simulink model "Diagrama de blocos - Matlab-SimulinkArquivo"  (R2019a)
settings: Solver=VariableStepAuto  StartTime=0.0  StopTime=15  RelTol=1e-6
libraries: simulink x1
settings Model: Creator=rcard  LastModifiedBy=rcard

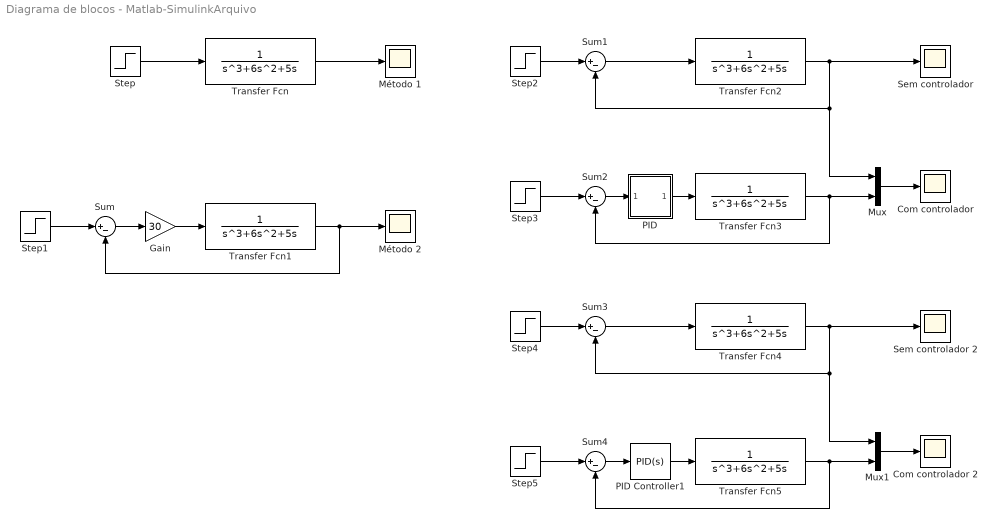
== system Diagrama de blocos - Matlab-SimulinkArquivo ==
  Com controlador : Scope
  Com controlador 2 : Scope
  Gain : Gain  Gain=30
  Mux : Mux  Inputs=2
  Mux1 : Mux  Inputs=2
  Método 1 : Scope
  Método 2 : Scope
  PID : Subsystem
  PID Controller1 : simulink/Continuous/PID Controller  Controller=PID  Form=Parallel  TimeDomain=Continuous-time  SampleTime=-1  IntegratorMethod=Forward Euler  FilterMethod=Forward Euler  ControllerParametersSource=internal  P=32.5  I=10.56  D=25  UseFilter=on  N=1000  TunerSelectOption=Transfer Function Based (PID Tuner App)  InitialConditionSource=internal  InitialConditionForIntegrator=0  InitialConditionForFilter=0  DifferentiatorICPrevScaledInput=0  ExternalReset=none  TrackingMode=off  Kt=1  LimitOutput=off  UpperSaturationLimit=inf  LowerSaturationLimit=-inf  LinearizeAsGain=on  AntiWindupMode=none  Kb=1  POutMin=[]  POutMax=[]  IOutMin=[]  IOutMax=[]  DOutMin=[]  DOutMax=[]  NOutMin=[]  NOutMax=[]  SumOutMin=[]  SumOutMax=[]  SaturationOutMin=[]  SaturationOutMax=[]  PParamMin=[]  PParamMax=[]  IParamMin=[]  IParamMax=[]  DParamMin=[]  DParamMax=[]  NParamMin=[]  NParamMax=[]  KbParamMin=[]  KbParamMax=[]  KtParamMin=[]  KtParamMax=[]  KbOutMin=[]  KbOutMax=[]  KtOutMin=[]  KtOutMax=[]  IntegratorOutMin=[]  IntegratorOutMax=[]  FilterOutMin=[]  FilterOutMax=[]  SumI1OutMin=[]  SumI1OutMax=[]  SumI2OutMin=[]  SumI2OutMax=[]  SumI3OutMin=[]  SumI3OutMax=[]  SumI4OutMin=[]  SumI4OutMax=[]  SumDOutMin=[]  SumDOutMax=[]  DifferentiatorOutMin=[]  DifferentiatorOutMax=[]  FilterDiffOutCoefMin=[]  FilterDiffOutCoefMax=[]  ReciprocalOutMin=[]  ReciprocalOutMax=[]  SumDenOutMin=[]  SumDenOutMax=[]  SumNumOutMin=[]  SumNumOutMax=[]  DivideOutMin=[]  DivideOutMax=[]  IntegratorContinuousStateAttributes=''  IntegratorStateMustResolveToSignalObject=off  IntegratorRTWStateStorageClass=Auto  FilterContinuousStateAttributes=''  FilterStateMustResolveToSignalObject=off  FilterRTWStateStorageClass=Auto  ParallelPVariant=InternalParameters  IdealPVariant=Disabled  IVariant=InternalParameters  DVariant=InternalParameters  IntegratorVariant=Continuous  SatVariant=Disabled  AWVariant=Passthrough  PCopyVariant=Disabled  TRVariant=Disabled  FdbkBlocksVariant=Forward  IdealPFdbkVariant=Disabled  SatFdbkVariant=Disabled  DerivativeFilterVariant=ContFilter  NVariant=InternalParameters  NCopyVariant=Disabled  FilterICVariant=InternalICsFilter  IntegratorICVariant=InternalICs  ExternalResetVariant=Disabled  TRSumVariant=Passthrough  SumFdbkVariant=Disabled  SumVariant=Sum_PID
  Sem controlador : Scope
  Sem controlador 2 : Scope
  Step{,1..5} (6 alike) : Step  Time=0  SampleTime=0
  Sum{,1..4} (5 alike) : Sum  Inputs=|+-
  Transfer Fcn{,1..5} (6 alike) : TransferFcn  Denominator="[1 6  5  0]"
  wires:
  Step1/1 -> Sum/1
  Sum/1 -> Gain/1
  Gain/1 -> Transfer Fcn1/1
  Transfer Fcn1/1 -> Sum/2, Método 2/1
  Transfer Fcn/1 -> Método 1/1
  Step/1 -> Transfer Fcn/1
  Step2/1 -> Sum1/1
  Transfer Fcn2/1 -> Mux/1, Sum1/2, Sem controlador/1
  Sum1/1 -> Transfer Fcn2/1
  Transfer Fcn3/1 -> Mux/2, Sum2/2
  Step3/1 -> Sum2/1
  Sum2/1 -> PID/1(In1)
  PID/1(Out1) -> Transfer Fcn3/1
  Mux/1 -> Com controlador/1
  Transfer Fcn4/1 -> Mux1/1, Sum3/2, Sem controlador 2/1
  Step5/1 -> Sum4/1
  Transfer Fcn5/1 -> Mux1/2, Sum4/2
  Sum3/1 -> Transfer Fcn4/1
  Mux1/1 -> Com controlador 2/1
  Sum4/1 -> PID Controller1/1
  PID Controller1/1 -> Transfer Fcn5/1
  Step4/1 -> Sum3/1

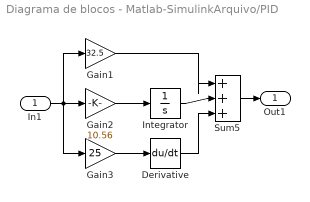
== system Diagrama de blocos - Matlab-SimulinkArquivo/PID ==
  In1 : Inport
  Derivative : Derivative
  Gain1 : Gain  Gain=32.5
  Gain2 : Gain  Gain=10.56
  Gain3 : Gain  Gain=25
  Integrator : Integrator
  Sum5 : Sum  Inputs=|+++
  Out1 : Outport
  wires:
  Gain2/1 -> Integrator/1
  Sum5/1 -> Out1/1
  Integrator/1 -> Sum5/2
  Gain1/1 -> Sum5/1
  Gain3/1 -> Derivative/1
  Derivative/1 -> Sum5/3
  In1/1 -> Gain3/1, Gain1/1, Gain2/1
